simulink model "simscape_SimpleMotorExample_20231124_0747"  (R2023b)
settings: Solver=ode23t  StartTime=0.0  StopTime=100  RelTol=1e-3
libraries: fl_lib x4, nesl_utility x3, ee_lib x3
settings Model: Creator=Patri  LastModifiedBy=Patri

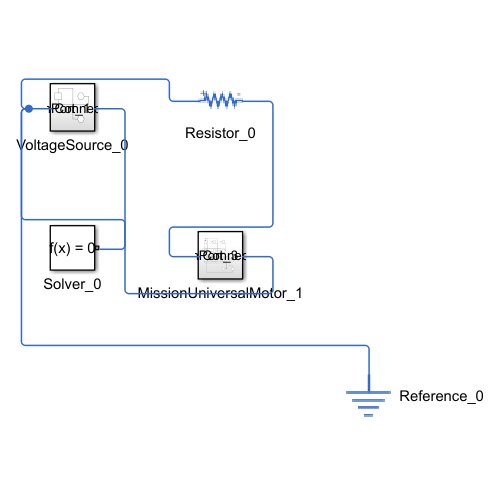
[thumbnail: Simulink's stored preview of the top-level diagram]
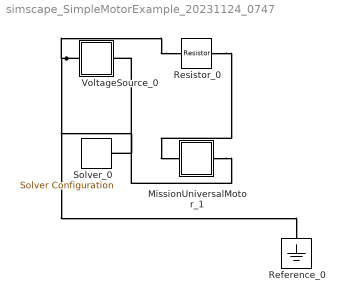
== system simscape_SimpleMotorExample_20231124_0747 ==
  MissionUniversalMotor_1 : Subsystem
  Reference_0 : fl_lib/Electrical/Electrical Elements/Electrical Reference
  Resistor_0 : ee_lib/Passive/Resistor  R=10.0 Ohm  enable_R_tol=ee.enum.toleranceApplication.none  R_tol=5  tol_distribution=ee.enum.toleranceDistribution.uniform  nSigma=4  enable_operating_limits=ee.enum.enable.no  operating_limit_action=ee.enum.passive.reportOpLim.warn  power_rating=1 W  max_working_voltage=100 V  enable_faults=ee.enum.enable.no  fault_action=simscape.enum.assert.action.none  R_faulted=inf Ohm  fault_trigger=ee.enum.faults.faultTrigger.temporal  t_fault=1 s  max_permissible_current=1 A  t_fail_on_current=1 s  noise_mode=ee.enum.sources.noise.Disabled  Tdevice=25 degC  sample_time=1e-3 s  repeatability=ee.enum.ic.repeatability.notRepeatable  user_seed=0  auto_seed=3890346746  faulted_specify=off  faulted_priority=None  faulted=0  power_derating_T1=70 degC  power_derating_T2=155 degC  operating_temperature_range_vec=[-50, 150] degC  alpha=3.93e-3 1/K  Tmeas=25 degC  thermal_mass=100 J/K  temperature_specify=off  temperature_priority=High  temperature=298.15 K  temperature_nominal_specify=off  temperature_nominal_unit=K  temperature_nominal_value=1
  Solver_0 : nesl_utility/Solver Configuration  PhysicalDomain=network_engine_domain  SubClassName=solver  LeftPortType=input  RightPortType=generic  Tones=[]  Harmonics=[]  SimulateNoise=off  Profile=off  UseLocalSampling=off  EnableSwitchedLinearOptims=on  FrequencyDomain=off  UseCCode=off  RelTol=0.001  AbsTol=0.001  MinStep=1e-09  ToWorkspace=off  RevertToSquareIcSolve=off  NumHomotopyIterations=100  PhasorMode=off  PhasorModeNumHarmonics=1  ConsistencySolver=NEWTON_XTOL_AFTER_FTOL  IndexReductionMethod=DerivativeReplacement  DoDC=off  ResidualTolerance=1e-09  ConsistencyTolSource=GLOBAL  ConsistencyAbsTol=0.001  ConsistencyRelTol=0.001  ConsistencyTolFactor=0.001  UseLocalSolver=off  LocalSolverChoice=NE_BACKWARD_EULER_ADVANCER  ResolveIndetEquations=on  FunctionEvalNumThread=1  LocalSolverSampleTime=0.001  DoFixedCost=off  MaxNonlinIter=3  MaxModeIter=2  ComputeImpulses=off  ImpulseIterations=2  LinearAlgebra=auto  LinearAlgebraNumThread=0  EquationFormulation=NE_TIME_EF  DelaysMemoryBudget=1024  AutomaticFiltering=on  FilteringTimeConstant=0.001  PartitionStorageMethod=AS_NEEDED  PartitionMemoryBudget=1024  PartitionMethod=ROBUST  MultibodyUseLocalSolver=off  MultibodyLocalSolverChoice=ODE1  MultibodyLocalSolverSampleTime=0.001
  VoltageSource_0 : Subsystem
  connections:
  Resistor_0/LConn1 -- VoltageSource_0/LConn1 -- Reference_0/LConn1 -- Solver_0/RConn1
  Resistor_0/RConn1 -- MissionUniversalMotor_1/LConn1
  MissionUniversalMotor_1/RConn1 -- VoltageSource_0/RConn1

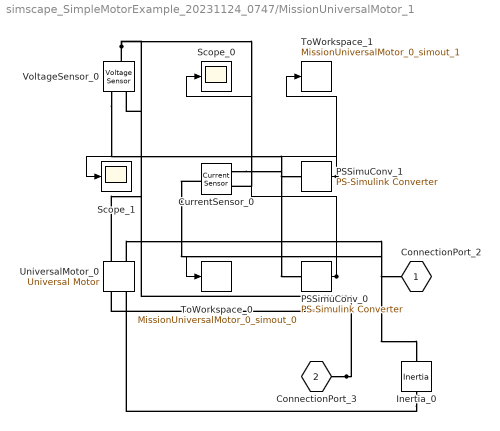
== system simscape_SimpleMotorExample_20231124_0747/MissionUniversalMotor_1 ==
  CurrentSensor_0 : fl_lib/Electrical/Electrical Sensors/Current Sensor
  Inertia_0 : fl_lib/Mechanical/Rotational Elements/Inertia  inertia=0.5 kg*m^2  num_ports=2.0  w_specify=off  w_priority=High  w=0 rad/s  w_nominal_specify=off  w_nominal_unit=rad/s  w_nominal_value=1  t_specify=off  t_priority=None  t=0 N*m  t_nominal_specify=off  t_nominal_unit=N*m  t_nominal_value=1
      settings: InternalSimscapePortConfiguration="{\"Bottom\":[],\"Left\":[{\"id\":\"I\",\"label\":\"\",\"type\":\"foundation.mechanical.rotational.rotational\"}],\"Right\":[{\"id\":\"J\",\"label\":\"\",\"type\":\"foundation.mechanical.rotational.rotational\"}],\"Top\":[]}"
  PSSimuConv_0 : nesl_utility/PS-Simulink Converter  PhysicalDomain=network_engine_domain  SubClassName=ps_output  LeftPortType=input  RightPortType=output  PseudoPeriodic=off  Frequencies=[]  VectorFormat=inherit  Unit=inherit  AffineConversion=off
  PSSimuConv_1 : nesl_utility/PS-Simulink Converter  PhysicalDomain=network_engine_domain  SubClassName=ps_output  LeftPortType=input  RightPortType=output  PseudoPeriodic=off  Frequencies=[]  VectorFormat=inherit  Unit=inherit  AffineConversion=off
  Scope_0 : Scope
  Scope_1 : Scope
  ToWorkspace_0 : ToWorkspace  VariableName=MissionUniversalMotor_0_simout_0  SaveFormat=Structure With Time  SampleTime=-1
  ToWorkspace_1 : ToWorkspace  VariableName=MissionUniversalMotor_0_simout_1  SaveFormat=Structure With Time  SampleTime=-1
  UniversalMotor_0 : ee_lib/Electromechanical/Brushed Motors/Universal Motor  parameterization=3  Ra=132.8 Ohm  Laf=0.1722 V*s/(A*rad)  w_rated=6500.0 rpm  P_rated=75.0 W  V_dc=200.0 V  T_max=0.39 N*m  P_in=160.0 W  V_ac=240 V  I_ac=0.8 A  w_ac=50 Hz  Ltot=0.525 H  J=2e-4 kg*m^2  lam=1e-6 N*m*s/rad  speed0=0 rpm  resistance_ratio=1  alpha=[.00393, .00393] 1/K  Tmeas=25 degC  thermal_masses=[100, 100] J/K  initial_temperatures=[25, 25] degC
      settings: InternalSimscapePortConfiguration="{\"Bottom\":[],\"Left\":[{\"id\":\"p\",\"label\":\"+\",\"type\":\"foundation.electrical.electrical\"},{\"id\":\"R\",\"label\":\"R\",\"type\":\"foundation.mechanical.rotational.rotational\"}],\"Right\":[{\"id\":\"n\",\"label\":\"-\",\"type\":\"foundation.electrical.electrical\"},{\"id\":\"C\",\"label\":\"C\",\"type\":\"foundation.mechanical.rotational.rotational\"}],\"Top\":[]}"
  VoltageSensor_0 : fl_lib/Electrical/Electrical Sensors/Voltage Sensor
  ConnectionPort_2 : PMIOPort  Side=Left
  ConnectionPort_3 : PMIOPort  Port=2  Side=Right
  wires:
  PSSimuConv_0/1 -> Scope_0/1, ToWorkspace_0/1
  PSSimuConv_1/1 -> Scope_1/1, ToWorkspace_1/1
  connections:
  CurrentSensor_0/LConn1 -- ConnectionPort_2/RConn1
  CurrentSensor_0/RConn2 -- VoltageSensor_0/LConn1 -- UniversalMotor_0/LConn1
  VoltageSensor_0/RConn2 -- ConnectionPort_3/RConn1 -- UniversalMotor_0/RConn1
  UniversalMotor_0/LConn2 -- Inertia_0/LConn1
  Inertia_0/RConn1 -- UniversalMotor_0/RConn2
  VoltageSensor_0/RConn1 -- PSSimuConv_0/LConn1
  CurrentSensor_0/RConn1 -- PSSimuConv_1/LConn1

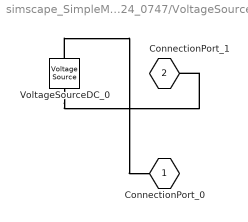
== system simscape_SimpleMotorExample_20231124_0747/VoltageSource_0 ==
  VoltageSourceDC_0 : ee_lib/Sources/Voltage Source  dc_voltage=10.0 V  ac_voltage=0 V  ac_shift=0 rad  ac_frequency=60 Hz  noise_mode=ee.enum.sources.noise.Disabled  PSD=0 V^2/Hz  sample_time=1e-3 s  repeatability=ee.enum.sources.repeatability.NotRepeatable  user_seed=0  auto_seed=3499211588  i_specify=off  i_priority=None  i=0 A  i_nominal_specify=off  i_nominal_unit=A  i_nominal_value=1  v_specify=off  v_priority=None  v=0 V  v_nominal_specify=off  v_nominal_unit=V  v_nominal_value=1
  ConnectionPort_0 : PMIOPort  Side=Left
  ConnectionPort_1 : PMIOPort  Port=2  Side=Right
  connections:
  VoltageSourceDC_0/LConn1 -- ConnectionPort_0/RConn1
  VoltageSourceDC_0/RConn1 -- ConnectionPort_1/RConn1
